simulink model "System_State_Observation_Simulation"  (Simulink 6.3)
settings: Solver=VariableStepDiscrete  StartTime=0.0  StopTime=100.0  RelTol=1e-3
libraries: simulink x1
settings Model: LastModifiedBy=Huang

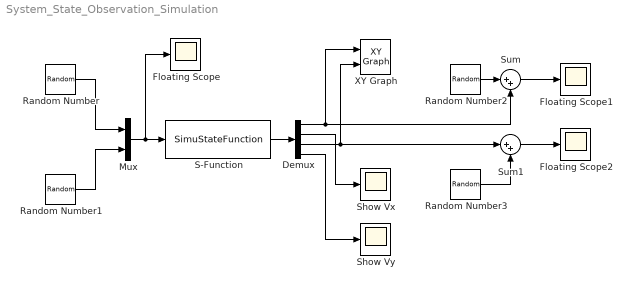
== system System_State_Observation_Simulation ==
  Demux : Demux
  Floating Scope : Scope
      settings: TimeRange=10  YMin=-3  YMax=2
  Floating Scope1 : Scope
      settings: SaveName=ScopeData3
  Floating Scope2 : Scope
      settings: SaveName=ScopeData4
  Mux : Mux  Description=Mux  Inputs=2
  Random Number : RandomNumber  Variance=0.01  SampleTime=1
  Random Number1 : RandomNumber  Variance=0.09  Seed=3  SampleTime=1
  Random Number2 : RandomNumber  Variance=0.04  Seed=34  SampleTime=1
  Random Number3 : RandomNumber  Variance=0.04  Seed=23  SampleTime=1
  S-Function : S-Function  FunctionName=SimuStateFunction
  Show Vx : Scope
  Show Vy : Scope
      settings: SaveName=ScopeData2
  Sum : Sum  Inputs=|++
  Sum1 : Sum  Inputs=|++
  XY Graph : simulink/Sinks/XY Graph  xmin=0  xmax=600  ymin=0  ymax=600  st=1
  wires:
  Random Number/1 -> Mux/1
  Random Number1/1 -> Mux/2
  Mux/1 -> Floating Scope/1, S-Function/1
  S-Function/1 -> Demux/1
  Demux/1 -> XY Graph/1, Sum/2
  Demux/3 -> XY Graph/2, Sum1/1
  Demux/4 -> Show Vy/1
  Demux/2 -> Show Vx/1
  Random Number2/1 -> Sum/1
  Random Number3/1 -> Sum1/2
  Sum/1 -> Floating Scope1/1
  Sum1/1 -> Floating Scope2/1
